simulink model "Sim_partie3"  (R2023b)
settings: Solver=FixedStepAuto  StartTime=0.0  StopTime=1000000  FixedStep=10  RelTol=1e-3
undefined symbols (not defined in the file): G, J2, Mt, phi, r, Rt, theta, v0
libraries: simulink x2
settings Model: Creator=louis  LastModifiedBy=louis

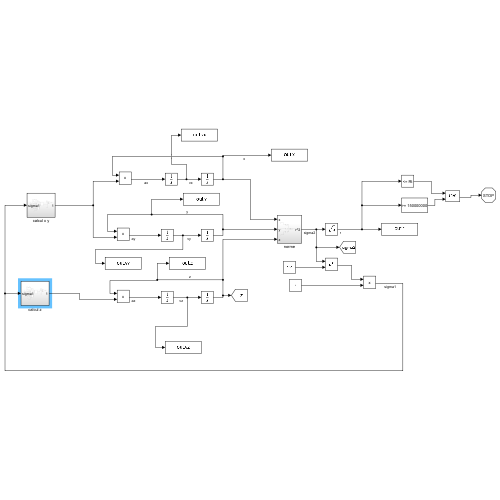
[thumbnail: Simulink's stored preview of the top-level diagram]
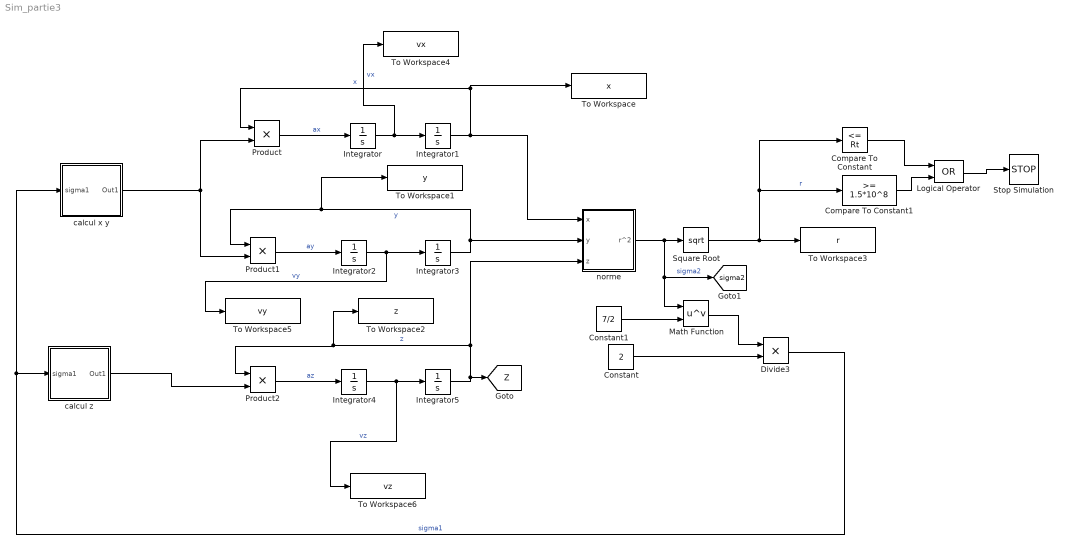
== system Sim_partie3 ==
  Compare To Constant : simulink/Logic and Bit Operations/Compare To Constant  relop=<=  const=Rt  OutDataTypeStr=boolean
  Compare To Constant1 : simulink/Logic and Bit Operations/Compare To Constant  relop=>=  const=1.5*10^8  OutDataTypeStr=boolean
  Constant : Constant  Value=2
  Constant1 : Constant  Value=7/2
  Divide3 : Product  Inputs=**
  Integrator : Integrator  InitialCondition=v0*sind(theta)
  Integrator1 : Integrator  InitialCondition=r*sind(phi)*cosd(theta)
  Integrator2 : Integrator  InitialCondition=-v0*cosd(theta)
  Integrator3 : Integrator  InitialCondition=r*sind(phi)*sind(theta)
  Integrator4 : Integrator
  Integrator5 : Integrator  InitialCondition=r*cosd(phi)
  Logical Operator : Logic  Operator=OR  AllPortsSameDT=off  OutDataTypeStr=boolean
  Math Function : Math  Operator=pow
  Product : Product
  Product1 : Product
  Product2 : Product
  Square Root : Sqrt
  Stop Simulation : Stop
  To Workspace : ToWorkspace  VariableName=x  SaveFormat=Timeseries  SampleTime=-1
  To Workspace1 : ToWorkspace  VariableName=y  SaveFormat=Timeseries  SampleTime=-1
  To Workspace2 : ToWorkspace  VariableName=z  SaveFormat=Timeseries  SampleTime=-1
  To Workspace3 : ToWorkspace  VariableName=r  SaveFormat=Timeseries  SampleTime=-1
  To Workspace4 : ToWorkspace  VariableName=vx  SaveFormat=Timeseries  SampleTime=-1
  To Workspace5 : ToWorkspace  VariableName=vy  SaveFormat=Timeseries  SampleTime=-1
  To Workspace6 : ToWorkspace  VariableName=vz  SaveFormat=Timeseries  SampleTime=-1
  calcul x y : Subsystem
  calcul z : Subsystem
  norme : Subsystem
  tag scope: Z=global, sigma2=global
  wires:
  Compare To Constant1/1 -> Logical Operator/2
  Product1/1 -> Integrator2/1  "ay"
  Compare To Constant/1 -> Logical Operator/1
  Integrator2/1 -> To Workspace5/1, Integrator3/1  "vy"
  Integrator4/1 -> To Workspace6/1, Integrator5/1  "vz"
  Integrator1/1 -> norme/1(x), Product/1, To Workspace/1  "x"
  Integrator5/1 -> [Z], norme/3(z), To Workspace2/1, Product2/1  "z"
  Product2/1 -> Integrator4/1  "az"
  Integrator/1 -> To Workspace4/1, Integrator1/1  "vx"
  Integrator3/1 -> Product1/1, To Workspace1/1, norme/2(y)  "y"
  Logical Operator/1 -> Stop Simulation/1
  Product/1 -> Integrator/1  "ax"
  norme/1(r^2) -> Square Root/1, [sigma2], Math Function/1  "sigma2"
  Square Root/1 -> Compare To Constant/1, Compare To Constant1/1, To Workspace3/1  "r"
  Constant/1 -> Divide3/2
  Math Function/1 -> Divide3/1
  Constant1/1 -> Math Function/2
  calcul x y/1(Out1) -> Product1/2, Product/2
  Divide3/1 -> calcul z/1(sigma1), calcul x y/1(sigma1)  "sigma1"
  calcul z/1(Out1) -> Product2/2

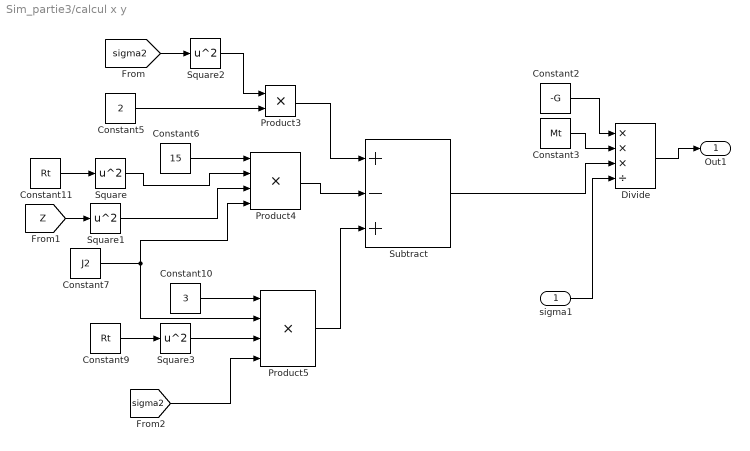
== system Sim_partie3/calcul x y ==
  sigma1 : Inport
  Constant10 : Constant  Value=3
  Constant11 : Constant  Value=Rt
  Constant2 : Constant  Value=-G
  Constant3 : Constant  Value=Mt
  Constant5 : Constant  Value=2
  Constant6 : Constant  Value=15
  Constant7 : Constant  Value=J2
  Constant9 : Constant  Value=Rt
  Divide : Product  Inputs=***/
  Product3 : Product
  Product4 : Product  Inputs=4
  Product5 : Product  Inputs=4
  Square{,1..3} (4 alike) : Math  Operator=square
  Subtract : Sum  Inputs=+-+
  Out1 : Outport
  wires:
  Constant7/1 -> Product5/2, Product4/4
  Constant6/1 -> Product4/1
  Square1/1 -> Product4/3
  Constant3/1 -> Divide/2
  Subtract/1 -> Divide/3
  Constant2/1 -> Divide/1
  Product3/1 -> Subtract/1
  Constant5/1 -> Product3/2
  Square/1 -> Product4/2
  Square2/1 -> Product3/1
  Product4/1 -> Subtract/2
  Constant11/1 -> Square/1
  Constant10/1 -> Product5/1
  Square3/1 -> Product5/3
  sigma1/1 -> Divide/4
  Constant9/1 -> Square3/1
  [sigma2] -> Product5/4
  [sigma2] -> Square2/1
  Product5/1 -> Subtract/3
  [Z] -> Square1/1
  Divide/1 -> Out1/1

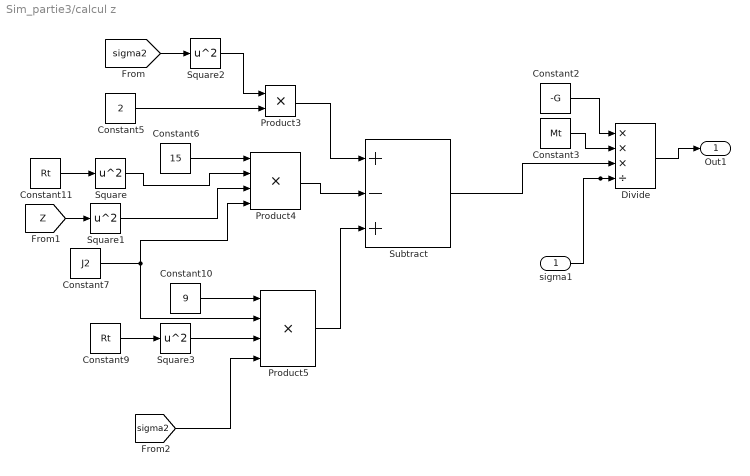
== system Sim_partie3/calcul z ==
  sigma1 : Inport
  Constant10 : Constant  Value=9
  Constant11 : Constant  Value=Rt
  Constant2 : Constant  Value=-G
  Constant3 : Constant  Value=Mt
  Constant5 : Constant  Value=2
  Constant6 : Constant  Value=15
  Constant7 : Constant  Value=J2
  Constant9 : Constant  Value=Rt
  Divide : Product  Inputs=***/
  Product3 : Product
  Product4 : Product  Inputs=4
  Product5 : Product  Inputs=4
  Square{,1..3} (4 alike) : Math  Operator=square
  Subtract : Sum  Inputs=+-+
  Out1 : Outport
  wires:
  Constant7/1 -> Product5/2, Product4/4
  Constant6/1 -> Product4/1
  Square1/1 -> Product4/3
  Constant3/1 -> Divide/2
  Subtract/1 -> Divide/3
  Constant2/1 -> Divide/1
  Product3/1 -> Subtract/1
  Constant5/1 -> Product3/2
  Square/1 -> Product4/2
  Square2/1 -> Product3/1
  Product4/1 -> Subtract/2
  Constant11/1 -> Square/1
  Constant10/1 -> Product5/1
  Square3/1 -> Product5/3
  sigma1/1 -> Divide/4
  Constant9/1 -> Square3/1
  [sigma2] -> Product5/4
  [sigma2] -> Square2/1
  Product5/1 -> Subtract/3
  [Z] -> Square1/1
  Divide/1 -> Out1/1

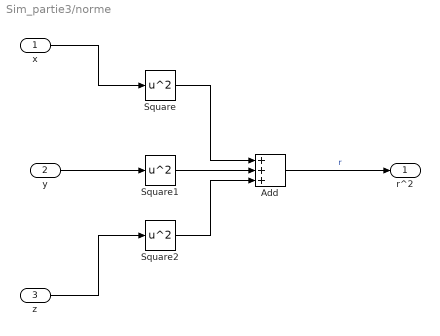
== system Sim_partie3/norme ==
  x : Inport
  y : Inport  Port=2
  z : Inport  Port=3
  Add : Sum  Inputs=+++
  Square : Math  Operator=square
  Square1 : Math  Operator=square
  Square2 : Math  Operator=square
  r^2 : Outport
  wires:
  x/1 -> Square/1
  Square2/1 -> Add/3
  Square1/1 -> Add/2
  Square/1 -> Add/1
  y/1 -> Square1/1
  z/1 -> Square2/1
  Add/1 -> r^2/1  "r"
